simulink model "am_demod_fixed_point_designer"  (R2021b)
settings: Solver=FixedStepAuto  StartTime=0.0  StopTime=20  RelTol=1e-3
libraries: commanapbnd3 x1, commchan3 x1
settings Model: DataTypeOverride=Off  MinMaxOverflowArchiveMode=Merge  FPTRunName=fxpOptimization.BaselineRun  Creator=caccolillo  LastModifiedBy=caccolillo
settings DataIOCC: SaveOutput=off  SaveTime=off
settings OptimizationCC: DefaultParameterBehavior=Inlined  UseDivisionForNetSlopeComputation=on  GainParamInheritBuiltInType=on  UseFloatMulNetSlope=on  InlineInvariantSignals=on  EfficientFloat2IntCast=on  LifeSpan=1
settings DebuggingCC: SignalRangeChecking=error  ParameterDowncastMsg=none  ParameterOverflowMsg=none  ParameterPrecisionLossMsg=none
settings HardwareCC: ProdLongLongMode=on
settings SFSimCC: MATLABDynamicMemAlloc=off
settings RTWCC: GenerateReport=on  LaunchReport=on
settings CodeAppCC: ForceParamTrailComments=on
settings GRTTargetCC: CombineSignalStateStructs=on  MatFileLogging=off  SupportVariableSizeSignals=on

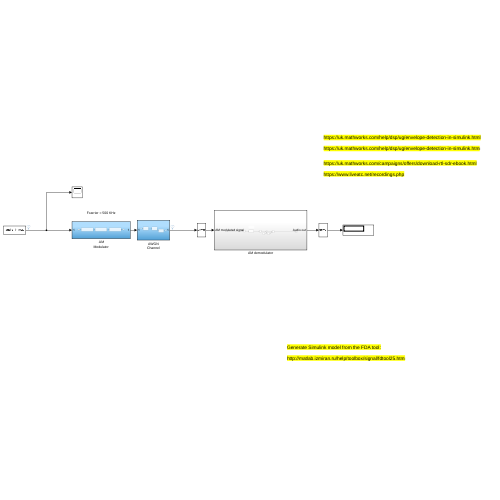
[thumbnail: Simulink's stored preview of the top-level diagram]
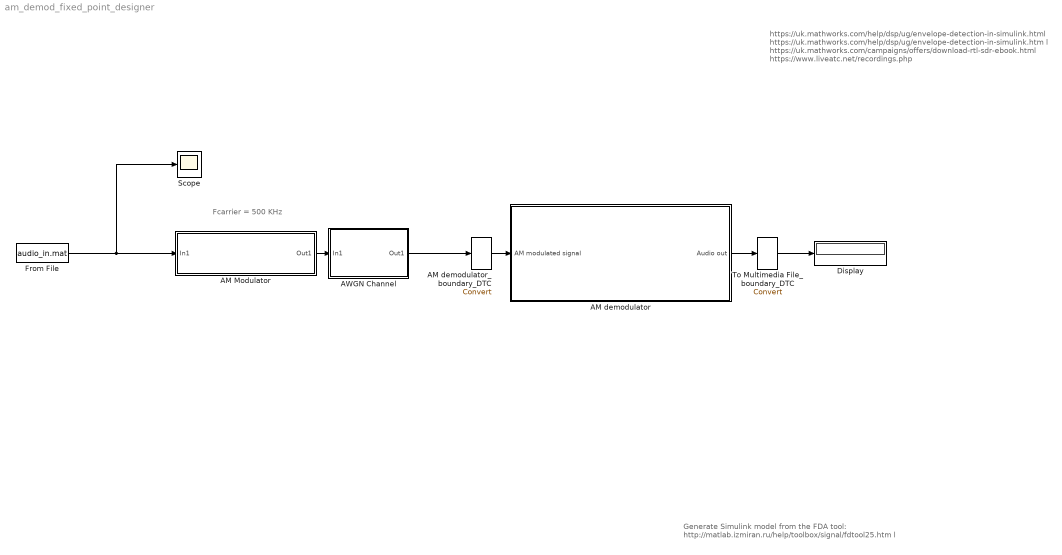
== system am_demod_fixed_point_designer ==
  note: Generate Simulink model from the FDA tool:
      |
      | http://matlab.izmiran.ru/help/toolbox/signal/fdtool25.htm l
  note: Fcarrier = 500 KHz
  note: https://uk.mathworks.com/help/dsp/ug/envelope-detection-in-simulink.html
      |
      | https://uk.mathworks.com/help/dsp/ug/envelope-detection-in-simulink.htm l
      |
      | https://uk.mathworks.com/campaigns/offers/download-rtl-sdr-ebook.html
      |
      | https://www.liveatc.net/recordings.php
  " AM Modulator " : Subsystem  Tag=DecoupledSystem
  AM demodulator : Subsystem
  AM demodulator_boundary_DTC : DataTypeConversion  SaturateOnIntegerOverflow=on  RndMeth=Zero
  AWGN Channel : Subsystem  Tag=DecoupledSystem
  Display : Display
  From File : FromFile  FileName=audio_in.mat  SampleTime=1/48000
  Scope : Scope
  To Multimedia File_boundary_DTC : DataTypeConversion  SaturateOnIntegerOverflow=on  RndMeth=Zero
  wires:
  From File/1 -> Scope/1, " AM Modulator "/1(In1)
  " AM Modulator "/1(Out1) -> AWGN Channel/1(In1)
  AWGN Channel/1(Out1) -> AM demodulator_boundary_DTC/1
  AM demodulator_boundary_DTC/1 -> AM demodulator/1(AM modulated signal)
  AM demodulator/1(Audio out) -> To Multimedia File_boundary_DTC/1
  To Multimedia File_boundary_DTC/1 -> Display/1

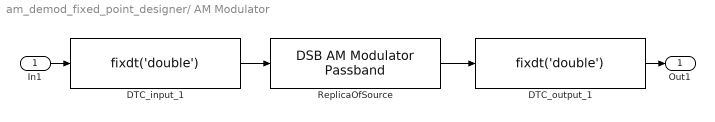
== system am_demod_fixed_point_designer/ AM Modulator  ==
  In1 : Inport  LockScale=on
  DTC_input_1 : DataTypeConversion  OutDataTypeStr=fixdt('double')  RndMeth=Nearest  LockScale=on
  DTC_output_1 : DataTypeConversion  OutDataTypeStr=fixdt('double')
  ReplicaOfSource : commanapbnd3/DSB AM Modulator Passband  Fc=500000  Ph=0  Offset=1
      settings: SourceProductBaseCode=CM
  Out1 : Outport  LockScale=on
  wires:
  In1/1 -> DTC_input_1/1
  DTC_input_1/1 -> ReplicaOfSource/1
  DTC_output_1/1 -> Out1/1
  ReplicaOfSource/1 -> DTC_output_1/1

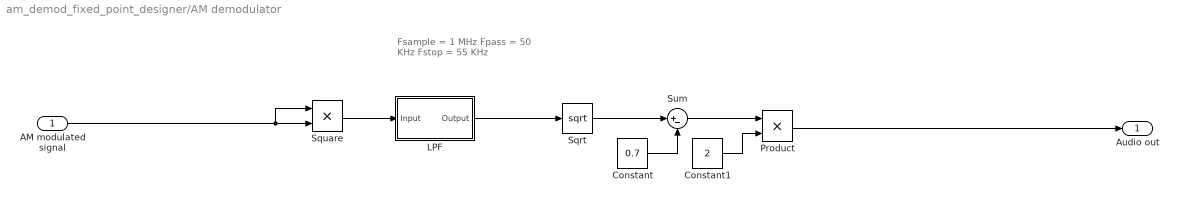
== system am_demod_fixed_point_designer/AM demodulator ==
  note: Fsample = 1 MHz
      | Fpass =  50 KHz
      | Fstop =  55 KHz
  AM modulated signal : Inport  OutMin=-2047  OutMax=2048
  Constant : Constant  Value=0.7  SampleTime=1e-6
  Constant1 : Constant  Value=2  SampleTime=1e-6
  LPF : Subsystem  Tag=FilterWizardSubSystem
      settings: ErrorFcn=dspFilterRealizedInBasicElemsAlgLoopErrFcnCallback
  Product : Product
  Sqrt : Sqrt  OutDataTypeStr=double  SaturateOnIntegerOverflow=on
  Square : Product
  Sum : Sum  Inputs=|+-
  Audio out : Outport  OutMin=-(2^15)-1  OutMax=2^15
  wires:
  Square/1 -> LPF/1(Input)
  Sqrt/1 -> Sum/1
  AM modulated signal/1 -> Square/1, Square/2
  Constant/1 -> Sum/2
  Sum/1 -> Product/1
  Constant1/1 -> Product/2
  LPF/1(Output) -> Sqrt/1
  Product/1 -> Audio out/1

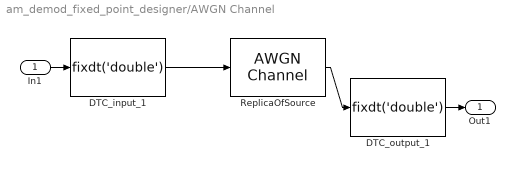
== system am_demod_fixed_point_designer/AWGN Channel ==
  In1 : Inport  LockScale=on
  DTC_input_1 : DataTypeConversion  OutDataTypeStr=fixdt('double')  RndMeth=Nearest  LockScale=on
  DTC_output_1 : DataTypeConversion  OutDataTypeStr=fixdt('double')
  ReplicaOfSource : commchan3/AWGN Channel  InputProcessing=Columns as channels (frame based)  seed=67  noiseMode="Signal to noise ratio  (Eb/No)"  EbNodB=75  EsNodB=10  SNRdB=10  bitsPerSym=1  Ps=1  Tsym=1  variance=1
  Out1 : Outport  LockScale=on
  wires:
  In1/1 -> DTC_input_1/1
  DTC_output_1/1 -> Out1/1
  DTC_input_1/1 -> ReplicaOfSource/1
  ReplicaOfSource/1 -> DTC_output_1/1

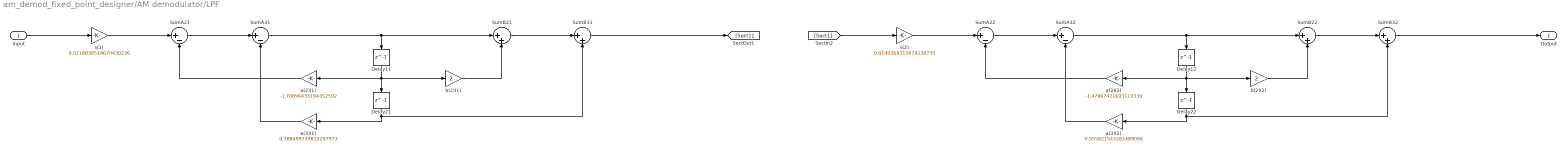
== system am_demod_fixed_point_designer/AM demodulator/LPF ==
  Input : Inport
  Delay{11..12,21..22} (4 alike) : Delay  DelayLength=1  InitialCondition=0
  SumA{21..22,31..32} (4 alike) : Sum  Inputs=|+-  OutDataTypeStr=double  RndMeth=Nearest  SaturateOnIntegerOverflow=on
  SumB{21..22,31..32} (4 alike) : Sum  Inputs=|++  OutDataTypeStr=double  RndMeth=Nearest  SaturateOnIntegerOverflow=on
  a(2)(1) : Gain  Gain=-1.70096433194352592  ParamDataTypeStr=double  OutDataTypeStr=double  RndMeth=Nearest  SaturateOnIntegerOverflow=on
  a(2)(2) : Gain  Gain=-1.47967421693119339  ParamDataTypeStr=double  OutDataTypeStr=double  RndMeth=Nearest  SaturateOnIntegerOverflow=on
  a(3)(1) : Gain  Gain=0.788499739815297973  ParamDataTypeStr=double  OutDataTypeStr=double  RndMeth=Nearest  SaturateOnIntegerOverflow=on
  a(3)(2) : Gain  Gain=0.555821543282489006  ParamDataTypeStr=double  OutDataTypeStr=double  RndMeth=Nearest  SaturateOnIntegerOverflow=on
  b(2)(1) : Gain  Gain=2  ParamDataTypeStr=double  OutDataTypeStr=double  RndMeth=Nearest  SaturateOnIntegerOverflow=on
  b(2)(2) : Gain  Gain=2  ParamDataTypeStr=double  OutDataTypeStr=double  RndMeth=Nearest  SaturateOnIntegerOverflow=on
  s(1) : Gain  Gain=0.0218838519679430236  ParamDataTypeStr=double  OutDataTypeStr=double  RndMeth=Nearest  SaturateOnIntegerOverflow=on
  s(2) : Gain  Gain=0.0190368315878238735  ParamDataTypeStr=double  OutDataTypeStr=double  RndMeth=Nearest  SaturateOnIntegerOverflow=on
  Output : Outport
  wires:
  Input/1 -> s(1)/1
  s(1)/1 -> SumA21/1
  SumA21/1 -> SumA31/1
  SumA31/1 -> SumB21/1, Delay11/1
  SumB21/1 -> SumB31/1
  SumB31/1 -> [Sect1]
  a(2)(1)/1 -> SumA21/2
  Delay11/1 -> a(2)(1)/1, b(2)(1)/1, Delay21/1
  b(2)(1)/1 -> SumB21/2
  a(3)(1)/1 -> SumA31/2
  Delay21/1 -> a(3)(1)/1, SumB31/2
  [Sect1] -> s(2)/1
  s(2)/1 -> SumA22/1
  SumA22/1 -> SumA32/1
  SumA32/1 -> SumB22/1, Delay12/1
  SumB22/1 -> SumB32/1
  SumB32/1 -> Output/1
  a(2)(2)/1 -> SumA22/2
  Delay12/1 -> a(2)(2)/1, b(2)(2)/1, Delay22/1
  b(2)(2)/1 -> SumB22/2
  a(3)(2)/1 -> SumA32/2
  Delay22/1 -> a(3)(2)/1, SumB32/2
